simulink model "Razor_StormSurge"  (R2021a)
settings: Solver=VariableStepAuto  StartTime=0.0  StopTime=10.0  RelTol=1e-3
values from neighbouring files (symbols this model uses):
  Av = 2.37    [loadVariables.m]
  Cd = 0.23    [loadVariables.m]
  Cr = 0.011    [loadVariables.m]
  g = 9.81    [loadVariables.m]
  mass = 1757.67    [loadVariables.m]
  MotSpdBrkPts = linspace(0, 837, 100)    [loadVariables.m]
  MotTrqPts = [MotTrqPts, Max_Mot_Trq]    [loadVariables.m]
  rho = 1.20    (= 1.2)    [loadVariables.m]
undefined symbols (not defined in the file or in its folder): Ki, P
libraries: autolibshared x1, pid_lib x1, autolibmotorctrlr x1, autolibpmsminterior x1, autolibinverter x1
settings Model: Creator=brand  LastModifiedBy=brand

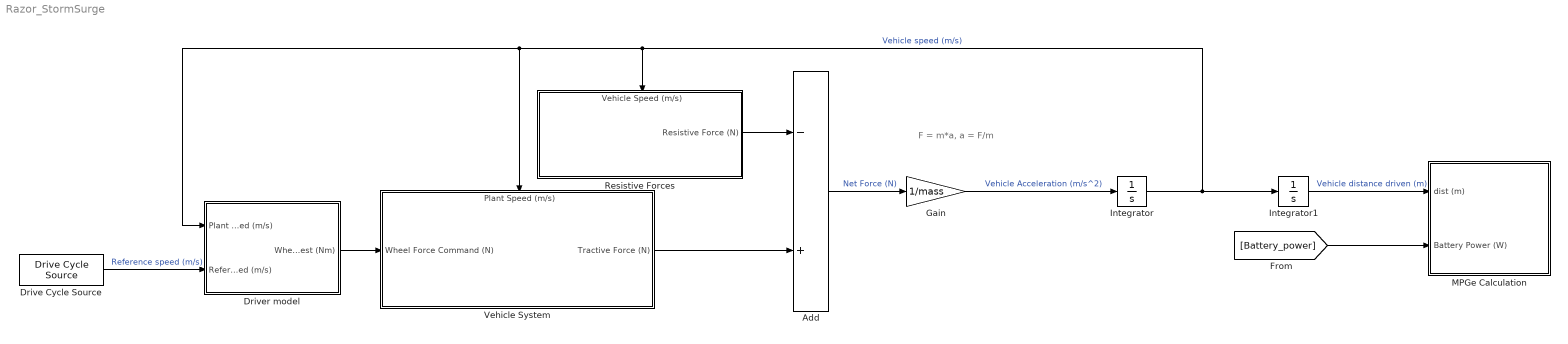
== system Razor_StormSurge ==
  note: F = m*a,
      | a = F/m
  Add : Sum  Inputs=-+
  Drive Cycle Source : autolibshared/Drive Cycle Source  cycleVar=UDDS  fileVar=cycleFTP75.mat  tfinal="1369  seconds, Cyclic"  cycleRepeat=on  outAccPort=off  outGearPort=off  gearList=No gear data  t_wot1=5  xdot_woto=0  xdot_wot1=30  t_wot2=20  xdot_wot2=0  t_wotend=30  srcUnit=m/s  outUnit=m/s  srcAccUnit=m/s/s  outAccUnit=m/s^2  dt=0  aMode=1  faultOption=off  velBnd=2  velBndUnit=mph  inUnit=m/s  timeBnd=1  failOption=off  stopSim=off  maxFaultCnt=10  maxFaultTime=2  maxTotFaultTime=15  traceOption=off  dtTrace=1  traceWindow=10  lastDCname=UDDS  lastOutUnit=mph  lastDT=0  lastTB=1  lastSB=2  forceCalcBound=off
      settings: SourceProductBaseCode=PW,DR,MT,UV,VE
  Driver model : Subsystem
  Gain : Gain  Gain=1/mass
  Integrator : Integrator
  Integrator1 : Integrator
  MPGe Calculation : Subsystem
  Resistive Forces : Subsystem
      settings: PortSchema="{\"entries\":[{\"content\":{\"sides\":[{\"content\":{\"connectorIds\":[]},\"type\":\"ConnectorPlacement.EquallySpacedRectSide\",\"uuid\":\"46fb1114-af3c-4ad6-a60f-2fe0fb91b046\"},{\"content\":{\"connectorIds\":[\"Out1\"],\"side\":\"RIGHT\"},\"type\":\"ConnectorPlacement.EquallySpacedRectSide\",\"uuid\":\"342c2ae1-b222-4ad6-a5d9-9f1c740209aa\"},{\"content\":{\"connectorIds\":[\"In1\"],\"side\":\"TOP\"},\"type\":\"ConnectorPlacement.EquallySpacedRectSide\",\"uuid\":\"3fbf4701-ba55-4f2a-97ae-f3f4d936c9ce\"}]},\"type\":\"ConnectorPlacement.EquallySpacedConnector\",\"uuid\":\"d737ea47-a616-4405-8433-a263aaccfb8a\"}],\"packageUris\":[\"http://schema.mathworks.com/mf0/Connector/R2020b\"],\"version\":\"1.0\"}"
  Vehicle System : Subsystem
      settings: PortSchema="{\"entries\":[{\"content\":{\"sides\":[{\"content\":{\"connectorIds\":[\"In1\"]},\"type\":\"ConnectorPlacement.EquallySpacedRectSide\",\"uuid\":\"abca09bb-aa9b-45d5-be79-2177664d57d3\"},{\"content\":{\"connectorIds\":[\"Out1\"],\"side\":\"RIGHT\"},\"type\":\"ConnectorPlacement.EquallySpacedRectSide\",\"uuid\":\"b4201239-485d-45a8-9291-64609474ff69\"},{\"content\":{\"connectorIds\":[\"In2\"],\"side\":\"TOP\"},\"type\":\"ConnectorPlacement.EquallySpacedRectSide\",\"uuid\":\"3a76b18e-21a7-440d-96f2-a8704a8317b2\"}]},\"type\":\"ConnectorPlacement.EquallySpacedConnector\",\"uuid\":\"d882d578-7c93-40cb-b2f2-49155aa3c911\"}],\"packageUris\":[\"http://schema.mathworks.com/mf0/Connector/R2020b\"],\"version\":\"1.0\"}"
  wires:
  Drive Cycle Source/1 -> Driver model/2(Reference speed (m/s))  "Reference speed (m/s)"
  Driver model/1(Wheel Force Request (Nm)) -> Vehicle System/1(Wheel Force Command (N))
  Resistive Forces/1(Resistive Force (N)) -> Add/1
  Vehicle System/1(Tractive Force (N)) -> Add/2
  Add/1 -> Gain/1  "Net Force (N)"
  Gain/1 -> Integrator/1  "Vehicle Acceleration (m/s^2)"
  Integrator/1 -> Driver model/1(Plant speed (m/s)), Vehicle System/2(Plant Speed (m/s)), Resistive Forces/1(Vehicle Speed (m/s)), Integrator1/1  "Vehicle speed (m/s)"
  Integrator1/1 -> MPGe Calculation/1(dist (m))  "Vehicle distance driven (m)"
  [Battery_power] -> MPGe Calculation/2(Battery Power (W))

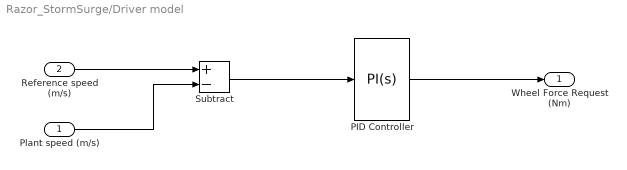
== system Razor_StormSurge/Driver model ==
  Plant speed (m/s) : Inport
  Reference speed (m/s) : Inport  Port=2
  PID Controller : pid_lib/PID Controller  Controller=PI  Form=Parallel  TimeDomain=Continuous-time  UseExternalTs=off  SampleTime=-1  IntegratorMethod=Forward Euler  FilterMethod=Forward Euler  ControllerParametersSource=internal  P=500  I=45  D=0  UseFilter=on  N=100  TunerSelectOption=Transfer Function Based (PID Tuner App)  InitialConditionSource=internal  InitialConditionForIntegrator=0  InitialConditionForFilter=0  DifferentiatorICPrevScaledInput=0  ExternalReset=none  TrackingMode=off  Kt=1  LimitOutput=off  SatLimitsSource=internal  UpperSaturationLimit=inf  LowerSaturationLimit=-inf  LinearizeAsGain=on  AntiWindupMode=none  Kb=1  POutMin=[]  POutMax=[]  IOutMin=[]  IOutMax=[]  DOutMin=[]  DOutMax=[]  NOutMin=[]  NOutMax=[]  SumOutMin=[]  SumOutMax=[]  SaturationOutMin=[]  SaturationOutMax=[]  PParamMin=[]  PParamMax=[]  IParamMin=[]  IParamMax=[]  DParamMin=[]  DParamMax=[]  NParamMin=[]  NParamMax=[]  KbParamMin=[]  KbParamMax=[]  KtParamMin=[]  KtParamMax=[]  KbOutMin=[]  KbOutMax=[]  KtOutMin=[]  KtOutMax=[]  IntegratorOutMin=[]  IntegratorOutMax=[]  FilterOutMin=[]  FilterOutMax=[]  SumI1OutMin=[]  SumI1OutMax=[]  SumI2OutMin=[]  SumI2OutMax=[]  SumI3OutMin=[]  SumI3OutMax=[]  SumI4OutMin=[]  SumI4OutMax=[]  SumDOutMin=[]  SumDOutMax=[]  DifferentiatorOutMin=[]  DifferentiatorOutMax=[]  FilterDiffOutCoefMin=[]  FilterDiffOutCoefMax=[]  ReciprocalOutMin=[]  ReciprocalOutMax=[]  SumDenOutMin=[]  SumDenOutMax=[]  SumNumOutMin=[]  SumNumOutMax=[]  DivideOutMin=[]  DivideOutMax=[]  UdiffTsProdOutMin=[]  UdiffTsProdOutMax=[]  NTsProdOutMin=[]  NTsProdOutMax=[]  UintegralTsProdOutMin=[]  UintegralTsProdOutMax=[]  UngainTsProdOutMin=[]  UngainTsProdOutMax=[]  IntegratorContinuousStateAttributes=''  IntegratorStateMustResolveToSignalObject=off  IntegratorRTWStateStorageClass=Auto  FilterContinuousStateAttributes=''  FilterStateMustResolveToSignalObject=off  FilterRTWStateStorageClass=Auto  ParallelPVariant=InternalParameters  IdealPVariant=Disabled  IVariant=InternalParameters  DVariant=Disabled  IntegratorVariant=Continuous  SatVariant=Disabled  AWVariant=Passthrough  PCopyVariant=Disabled  TRVariant=Disabled  FdbkBlocksVariant=Forward  IdealPFdbkVariant=Disabled  SatFdbkVariant=Disabled  DerivativeFilterVariant=Disabled  NVariant=Disabled  NCopyVariant=Disabled_SignalSpec  FilterICVariant=Disabled  IntegratorICVariant=InternalICs  ExternalResetVariant=Disabled  TRSumVariant=Passthrough  SumFdbkVariant=Disabled  SumVariant=Sum_PI  TsampFilterVariant=InternalTs  TsampNgainVariant=Passthrough  TsampIntegralVariant=Passthrough  ExternalSaturationOutDataTypeStr=Inherit: Same as second input
  Subtract : Sum  Inputs=+-
  Wheel Force Request (Nm) : Outport
  wires:
  Reference speed (m/s)/1 -> Subtract/1
  Plant speed (m/s)/1 -> Subtract/2
  Subtract/1 -> PID Controller/1
  PID Controller/1 -> Wheel Force Request (Nm)/1

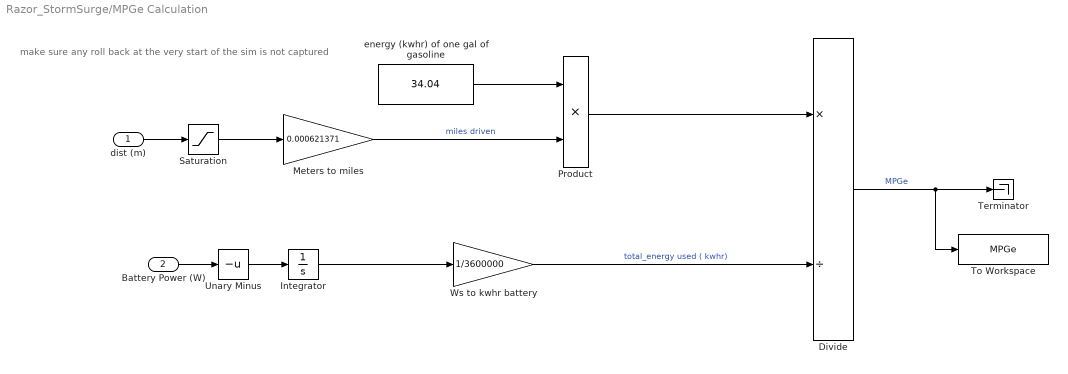
== system Razor_StormSurge/MPGe Calculation ==
  note: make sure any roll back at the very start of the sim is not captured
  dist (m) : Inport
  Battery Power (W) : Inport  Port=2
  Divide : Product  Inputs=*/
  Integrator : Integrator
  Meters to miles : Gain  Gain=0.000621371
  Product : Product
  Saturation : Saturate  UpperLimit=inf  LowerLimit=0
  Terminator : Terminator
  To Workspace : ToWorkspace  VariableName=MPGe  SaveFormat=Timeseries  SampleTime=-1
  Unary Minus : UnaryMinus
  Ws to kwhr battery : Gain  Gain=1/3600000
  energy (kwhr) of one gal of gasoline : Constant  Value=34.04
  wires:
  dist (m)/1 -> Saturation/1
  Battery Power (W)/1 -> Unary Minus/1
  Integrator/1 -> Ws to kwhr battery/1
  Ws to kwhr battery/1 -> Divide/2  "total_energy used ( kwhr)"
  Meters to miles/1 -> Product/2  "miles driven"
  energy (kwhr) of one gal of gasoline/1 -> Product/1
  Product/1 -> Divide/1
  Divide/1 -> To Workspace/1, Terminator/1  "MPGe"
  Saturation/1 -> Meters to miles/1
  Unary Minus/1 -> Integrator/1

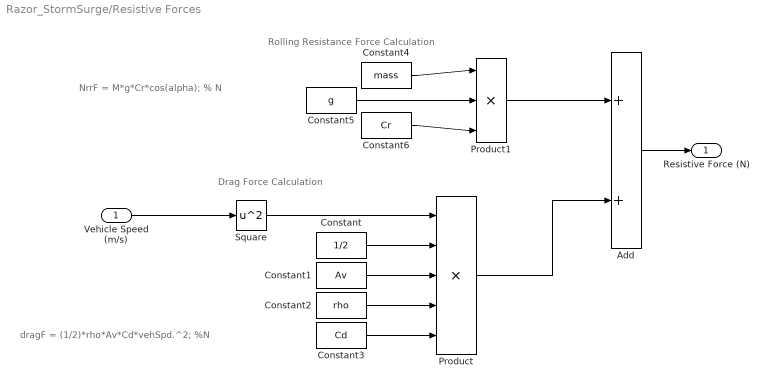
== system Razor_StormSurge/Resistive Forces ==
  note: dragF = (1/2)*rho*Av*Cd*vehSpd.^2; %N
  note: Rolling Resistance Force Calculation
  note: Drag Force Calculation
  note: NrrF = M*g*Cr*cos(alpha); % N
  Vehicle Speed (m/s) : Inport
  Add : Sum
  Constant : Constant  Value=1/2
  Constant1 : Constant  Value=Av
  Constant2 : Constant  Value=rho
  Constant3 : Constant  Value=Cd
  Constant4 : Constant  Value=mass
  Constant5 : Constant  Value=g
  Constant6 : Constant  Value=Cr
  Product : Product  Inputs=5
  Product1 : Product  Inputs=3
  Square : Math  Operator=square  SaturateOnIntegerOverflow=on
  Resistive Force (N) : Outport
  wires:
  Add/1 -> Resistive Force (N)/1
  Vehicle Speed (m/s)/1 -> Square/1
  Square/1 -> Product/1
  Constant/1 -> Product/2
  Constant3/1 -> Product/5
  Constant2/1 -> Product/4
  Constant1/1 -> Product/3
  Product/1 -> Add/2
  Product1/1 -> Add/1
  Constant4/1 -> Product1/1
  Constant6/1 -> Product1/3
  Constant5/1 -> Product1/2

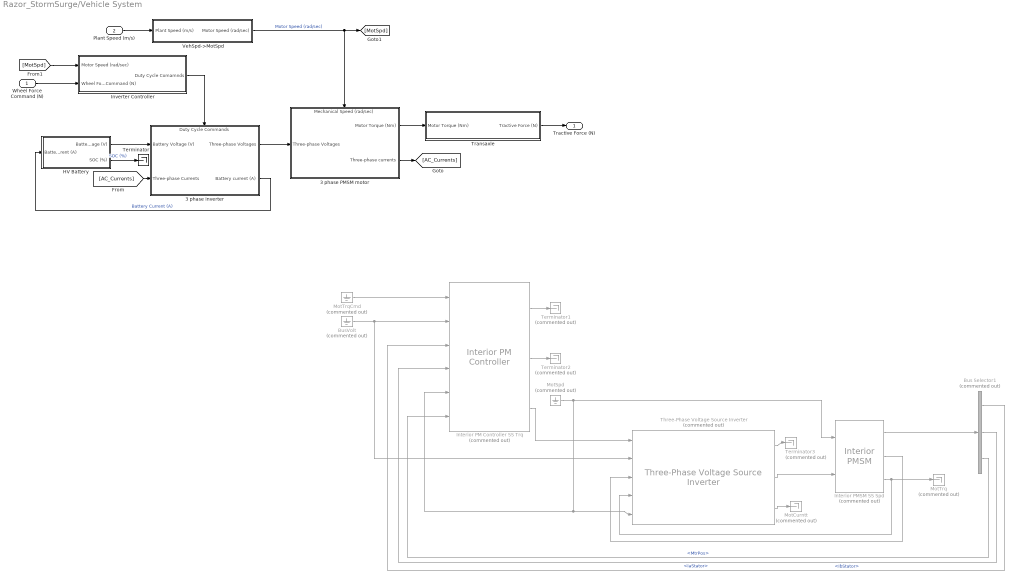
== system Razor_StormSurge/Vehicle System ==
  Wheel Force Command (N) : Inport
  Plant Speed (m/s) : Inport  Port=2
  3 phase PMSM motor : Subsystem
      settings: PortSchema="{\"entries\":[{\"content\":{\"sides\":[{\"content\":{\"connectorIds\":[\"In1\"]},\"type\":\"ConnectorPlacement.EquallySpacedRectSide\",\"uuid\":\"126b70eb-255c-48da-b14a-59d51f4de6ab\"},{\"content\":{\"connectorIds\":[\"Out1\",\"Out2\"],\"side\":\"RIGHT\"},\"type\":\"ConnectorPlacement.EquallySpacedRectSide\",\"uuid\":\"d32f0671-953a-483c-9d61-f5cd187321ce\"},{\"content\":{\"connectorIds\":[\"In2\"],\"side\":\"TOP\"},\"type\":\"ConnectorPlacement.EquallySpacedRectSide\",\"uuid\":\"eb86438b-ec89-4301-94d8-73a9bc17eed4\"}]},\"type\":\"ConnectorPlacement.EquallySpacedConnector\",\"uuid\":\"154c2a3e-5c55-43f0-9c3b-679d71a84e64\"}],\"packageUris\":[\"http://schema.mathworks.com/mf0/Connector/R2020b\"],\"version\":\"1.0\"}"
  3 phase inverter : Subsystem
      settings: PortSchema="{\"entries\":[{\"content\":{\"sides\":[{\"content\":{\"connectorIds\":[\"In1\",\"In2\"]},\"type\":\"ConnectorPlacement.EquallySpacedRectSide\",\"uuid\":\"4a21ea7b-e427-4998-a010-d9c8d20698f5\"},{\"content\":{\"connectorIds\":[\"Out1\",\"Out2\"],\"side\":\"RIGHT\"},\"type\":\"ConnectorPlacement.EquallySpacedRectSide\",\"uuid\":\"8123b628-bceb-4e34-b96a-055da3824839\"},{\"content\":{\"connectorIds\":[\"In3\"],\"side\":\"TOP\"},\"type\":\"ConnectorPlacement.EquallySpacedRectSide\",\"uuid\":\"dfcbad7e-f150-4406-9c78-1ff00b62013a\"}]},\"type\":\"ConnectorPlacement.EquallySpacedConnector\",\"uuid\":\"e87e79eb-e09f-4775-b20f-06c8dce35028\"}],\"packageUris\":[\"http://schema.mathworks.com/mf0/Connector/R2020b\"],\"version\":\"1.0\"}"
  Bus Selector1 : BusSelector  Commented=on  OutputSignals=IaStator,IbStator,MtrPos
  BusVolt : Ground  Commented=on
  HV Battery : Subsystem
  Interior PM Controller SS Trq : autolibmotorctrlr/Interior PM Controller  Commented=on  control_type=Torque Control  Rs=Rs  Ld=Ld  Lq=Lq  lambda_pm=lambda_pm  PolePairs=PolePairs  Mechanical=Mechanical  T_max=T_max  bp=10  T_mtpa=T_mtpa  id_mtpa=id_mtpa  iq_mtpa=iq_mtpa  idq_limits=idq_limits  EV_current=EV_current  Tst=5e-5  Kp_d=Kp_d  Kp_q=Kp_q  Ki=Ki  EV_motion=EV_motion  EV_sf=EV_sf  ba=ba  Ksa=Ksa  Kisa=Kisa  Ksf=Ksf  Jcomp=Jcomp  Fv=Fv  Fs=Fs  param_loss=Single efficiency measurement  eff=98  w_loss_bp=[0 200 400 600 800 1000]  T_loss_bp=[0 25 50 75 100]  losses_table=[100 100 100 100 100;100 150 200 250 300;100 200 300 400 500;100 250 400 550 700;100 300 500 700 900;100 350 600 850 1100]  w_eff_bp=[200 400 600 800 1000]  T_eff_bp=[25 50 75 100]  efficiency_table=[96.2 98.1 98.7 99;98.1 99 99.4 99.5;98.7 99.4 99.6 99.7;99 99.5 99.7 99.8;99.2 99.6 99.7 99.8]  x_w_bp=[-1000 -800 -600 -400 -200 200 400 600 800 1000]  x_T_bp=[-100 -75 -50 -25 25 50 75 100]  x_losses_mat=[200.400801603196 225.67703109328 200.803212851408 201.612903225806 199.999999999997 200 225 200;160.320641282556 180.541624874624 201.005025125625 202.020202020203 200 200 180 160;180.541624874624 180.722891566267 181.086519114686 197.568389057748 194.999999999999 179.999999999997 180 180;201.005025125625 181.086519114686 202.020202020203 193.67991845056 190 200 179.999999999997 200;202.020202020203 197.568389057748 193.67991845056 197.505197505197 190 190 194.999999999999 200;200 194.999999999999 190 190 197.505197505197 193.67991845056 197.568389057748 202.020202020203;200 179.999999999997 200 190 193.67991845056 202.020202020203 181.086519114686 201.005025125625;180 180 179.999999999997 194.999999999999 197.568389057748 181.086519114686 180.722891566267 180.541624874624;160 180 200 200 202.020202020203 201.005025125625 180.541624874624 160.320641282556;200 225 200 199.999999999997 201.612903225806 200.803212851408 225.67703109328 200.400801603196]  Tsm=5e-4
      settings: SourceProductBaseCode=PW
  Interior PMSM SS Spd : autolibpmsminterior/Interior PMSM  Commented=on  port_config=Speed  sim_type=Continuous  Ts=0.001  P=P  Rs=Rs  Ldq=Ldq  KConstText=Permanent flux linkage constant (lambda_pm):  lambda_pm=lambda_pm  Ke=159.9771  mechanical=mechanical  idq0=idq0  theta_init=theta_init  omega_init=omega_init  KConst=lambda_pm  lambda_pm_calc=lambda_pm  Kt=1.323  RefBlkName='autolibpmsminterior/Interior PMSM'  aMode=1
      settings: SourceProductBaseCode=PW,DR,MT,UV,VE
  Inverter Controller : Subsystem
  MotCurntt : Terminator  Commented=on
  MotSpd : Ground  Commented=on
  MotTrq : Terminator  Commented=on
  MotTrqCmd : Ground  Commented=on
  Terminator : Terminator
  Terminator1 : Terminator  Commented=on
  Terminator2 : Terminator  Commented=on
  Terminator3 : Terminator  Commented=on
  Three-Phase Voltage Source Inverter : autolibinverter/Three-Phase Voltage Source Inverter  Commented=on  InvrtrTmpInpEnbl=off  enable_hdl=off  model_type=Commanded phase voltage  fs=5000  w_eff_bp=[-1000 -500 0 500 1000]  n1=128  T_eff_bp=[-200 -100 0 100 200]  Temp_eff_bp=[213.15 293.15 373.15]  n2=128  ploss_table=0.98*ones(5,5)  ploss_table_3d=cat(3,0.95*[1 0.999 0.989 0.997 0.996;0.995 0.994 0.993 0.992 0.991;0.990 0.989 0.988 0.987 0.986;0.985 0.984 0.983 0.982 0.981;0.980 0.979 0.978 0.977 0.976],[1 0.999 0.989 0.997 0.996;0.995 0.994 0.993 0.992 0.991;0.990 0.989 0.988 0.987 0.986;0.985 0.984 0.983 0.982 0.981;0.980 0.979 0.978 0.977 0.976],0.92*[1 0.999 0.989 0.997 0.996;0.995 0.994 0.993 0.992 0.991;0.990 0.989 0.988 0.987 0.986;0.985 0.984 0.983 0.982 0.981;0.980 0.979 0.978 0.977 0.976])  preExtrapFlag=off  u1max=1000  u1min=-1000  u2max=200  u2min=-200  intPrec=23  RefBlkName='autolibmappedmotor/Mapped Motor'  CalLossMapData={}  CalLossWithTempMapData={}
      settings: SourceProductBaseCode=PW,DR,MT,UV,VE
  Transaxle : Subsystem
  VehSpd->MotSpd : Subsystem
  Tractive Force (N) : Outport
  wires:
  HV Battery/1(Battery Voltage (V)) -> 3 phase inverter/1(Battery Voltage (V))
  3 phase inverter/2(Battery current (A)) -> HV Battery/1(Battery Current (A))  "Battery Current (A)"
  3 phase inverter/1(Three-phase Voltages) -> 3 phase PMSM motor/1(Three-phase Voltages)
  3 phase PMSM motor/2(Three-phase currents) -> [AC_Currents]
  [AC_Currents] -> 3 phase inverter/2(Three-phase Currents)
  3 phase PMSM motor/1(Motor Torque (Nm)) -> Transaxle/1(Motor Torque (Nm))
  Transaxle/1(Tractive Force (N)) -> Tractive Force (N)/1
  HV Battery/2(SOC (%)) -> Terminator/1  "SOC (%)"
  Inverter Controller/1(Duty Cycle Comamnds) -> 3 phase inverter/3(Duty Cycle Commands)
  Wheel Force Command (N)/1 -> Inverter Controller/2(Wheel Force Command (N))
  Plant Speed (m/s)/1 -> VehSpd->MotSpd/1(Plant Speed (m/s))
  VehSpd->MotSpd/1(Motor Speed (rad/sec)) -> [MotSpd], 3 phase PMSM motor/2(Mechanical Speed (rad/sec))  "Motor Speed (rad/sec)"
  [MotSpd] -> Inverter Controller/1(Motor Speed (rad/sec))
  Interior PMSM SS Spd/3 -> MotTrq/1, Three-Phase Voltage Source Inverter/4
  Interior PM Controller SS Trq/3 -> Three-Phase Voltage Source Inverter/1
  Three-Phase Voltage Source Inverter/3 -> MotCurntt/1
  Interior PMSM SS Spd/2 -> Three-Phase Voltage Source Inverter/3
  Interior PM Controller SS Trq/1 -> Terminator1/1
  Three-Phase Voltage Source Inverter/2 -> Interior PMSM SS Spd/2
  MotSpd/1 -> Interior PMSM SS Spd/1, Three-Phase Voltage Source Inverter/5, Interior PM Controller SS Trq/5
  BusVolt/1 -> Three-Phase Voltage Source Inverter/2, Interior PM Controller SS Trq/2
  Bus Selector1/1 -> Interior PM Controller SS Trq/3  "<IaStator>"
  Interior PM Controller SS Trq/2 -> Terminator2/1
  Bus Selector1/3 -> Interior PM Controller SS Trq/6  "<MtrPos>"
  Bus Selector1/2 -> Interior PM Controller SS Trq/4  "<IbStator>"
  Interior PMSM SS Spd/1 -> Bus Selector1/1
  Three-Phase Voltage Source Inverter/1 -> Terminator3/1
  MotTrqCmd/1 -> Interior PM Controller SS Trq/1

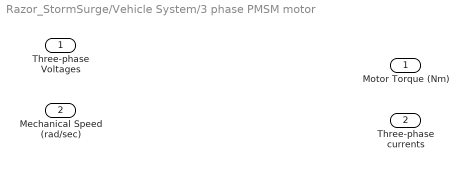
== system Razor_StormSurge/Vehicle System/3 phase PMSM motor ==
  Three-phase Voltages : Inport
  Mechanical Speed (rad/sec) : Inport  Port=2
  Motor Torque (Nm) : Outport
  Three-phase currents : Outport  Port=2

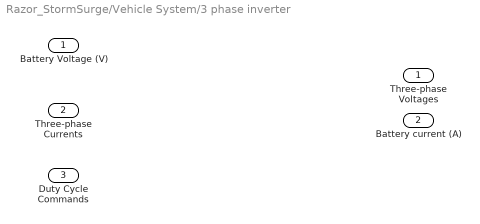
== system Razor_StormSurge/Vehicle System/3 phase inverter ==
  Battery Voltage (V) : Inport
  Three-phase Currents : Inport  Port=2
  Duty Cycle Commands : Inport  Port=3
  Three-phase Voltages : Outport
  Battery current (A) : Outport  Port=2

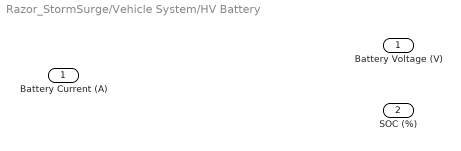
== system Razor_StormSurge/Vehicle System/HV Battery ==
  Battery Current (A) : Inport
  Battery Voltage (V) : Outport
  SOC (%) : Outport  Port=2

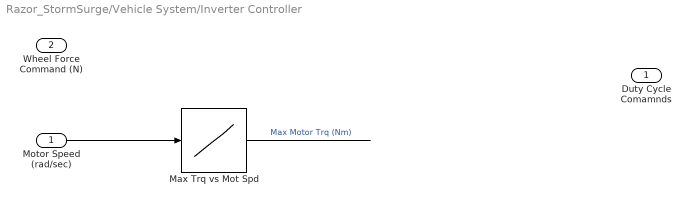
== system Razor_StormSurge/Vehicle System/Inverter Controller ==
  Motor Speed (rad/sec) : Inport
  Wheel Force Command (N) : Inport  Port=2
  Max Trq vs Mot Spd : Lookup_n-D  NumberOfTableDimensions=1  BreakpointsForDimension1=MotSpdBrkPts  Table=MotTrqPts  InternalRulePriority=Speed  RndMeth=Simplest  InputSameDT=on
  Duty Cycle Comamnds : Outport
  wires:
  Motor Speed (rad/sec)/1 -> Max Trq vs Mot Spd/1
  Max Trq vs Mot Spd/1 -> ?  "Max Motor Trq (Nm)"

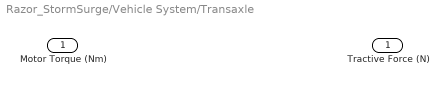
== system Razor_StormSurge/Vehicle System/Transaxle ==
  Motor Torque (Nm) : Inport
  Tractive Force (N) : Outport

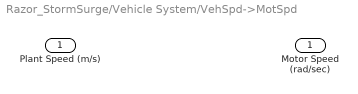
== system Razor_StormSurge/Vehicle System/VehSpd->MotSpd ==
  Plant Speed (m/s) : Inport
  Motor Speed (rad/sec) : Outport
